simulink model "ModelNonLinearMechFram"  (R2014b)
settings: Solver=ode45  StartTime=0.0  StopTime=1.5  FixedStep=0.001  RelTol=1e-3
InitFcn:
  | InitModel;
values from neighbouring files (symbols this model uses):
  R1 = 1.8e3    (= 1800)    [InitModel.m]    (also in SystemModel.m; SystemModel_marco.m)
  R4 = 47e3    (= 47000)    [InitModel.m]    (also in SystemModel.m; SystemModel_marco.m)
  R6 = 100e3    (= 100000)    [InitModel.m]    (also in SystemModel.m; SystemModel_marco.m)
  R7 = 27e3    (= 27000)    [InitModel.m]    (also in SystemModel.m; SystemModel_marco.m)
  rad2rpm = 60/(2*pi)    (= 9.54929658551)    [InitModel.m]    (also in SystemModel.m)
  Rs = 0.1    [InitModel.m]    (also in SystemModel.m; SystemModel_marco.m)
  Rv2 = realp('Rv2', 0)    [InitModel.m]    (also in SystemModel.m = realp('Rv2', 10000); SystemModel_marco.m = 0)
  Vdc = 30/8    (= 3.75)    [InitModel.m]    (also in SystemModel.m = 30; SystemModel_marco.m = 30)
  Vsat = 10    [InitModel.m]
undefined symbols (not defined in the file or in its folder): motor, pid, sigbuilder_block
libraries: cstblocks x5, simulink x1
settings Model: Creator=Edoardo  LastModifiedBy=Edoardo
settings SolverCC: ZeroCrossAlgorithm=Adaptive

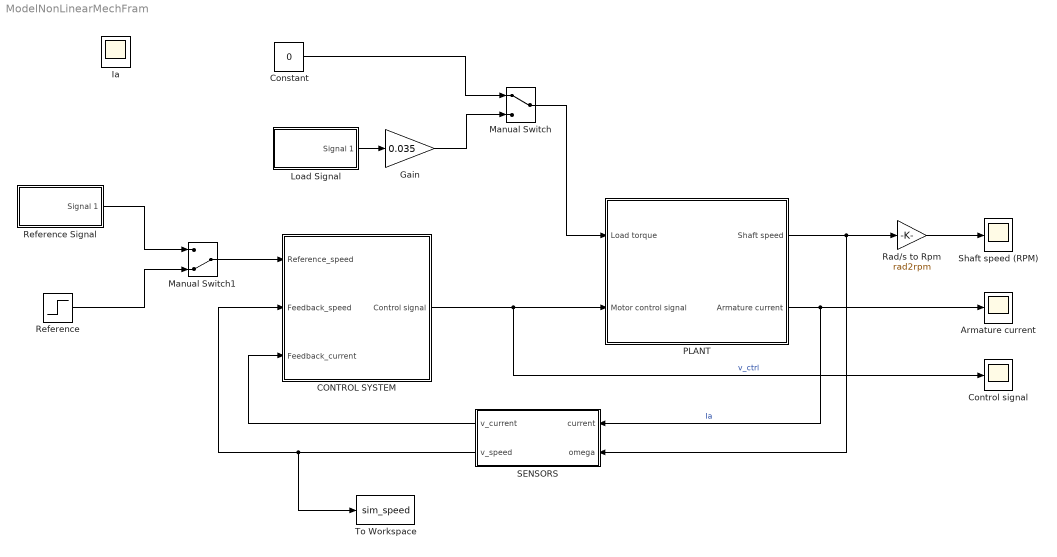
== system ModelNonLinearMechFram ==
  "Armature current " : Scope
      settings: YMin=-0.2  YMax=1.4  SaveName=ScopeData3
  CONTROL SYSTEM : Subsystem
  Constant : Constant  Value=0
  Control signal : Scope
      settings: YMin=-0.2  YMax=1.4  SaveName=ScopeData5
  Gain : Gain  Gain=0.035
  Load Signal : Subsystem  Tag=STV Subsys  LoadFcn=sigbuilder_block('load');  StartFcn=sigbuilder_block('start');  StopFcn=sigbuilder_block('stop');  ClipboardFcn=sigbuilder_block('clipboard');  mask(Sigbuilder block){}
      mask help: Simulink:masks:SigbuilderBlock_MD
      mask init:
      | if ~strcmp(get_param(bdroot(gcbh),'SimulationStatus'),'stopped') tuvar = sigbuilder_block('maskInit'); end
      settings: CopyFcn=sigbuilder_block('copy');  DeleteFcn=sigbuilder_block('delete');  ModelCloseFcn=sigbuilder_block('modelClose');  PreSaveFcn=sigbuilder_block('preSave');  PauseFcn=sigbuilder_block('pause');  ContinueFcn=sigbuilder_block('continue');  NameChangeFcn=sigbuilder_block('namechange');  OpenFcn=sigbuilder_block('open',[437.6 199.2 550.4 400 ]);  CloseFcn=sigbuilder_block('close');
      mask Display: plot(0, 0, 100, 100,[2, 2, 32, 32, 2], [68, 8, 8, 68, 68],[32, 2], [38, 38], [32, 19, 2],[53, 60, 44], [32, 17, 17, 2],[16, 16, 31, 31]);txt = getActiveGroup(gcbh);text(2, 100, txt,'verticalAlignment', 'top');
  Manual Switch : ManualSwitch
  Manual Switch1 : ManualSwitch  CurrentSetting=0
  PLANT : Subsystem
  Rad/s to Rpm : Gain  Gain=rad2rpm
  Reference : Step  Time=0.5  After=8  SampleTime=0
  Reference Signal : Subsystem  Tag=STV Subsys  LoadFcn=sigbuilder_block('load');  StartFcn=sigbuilder_block('start');  StopFcn=sigbuilder_block('stop');  ClipboardFcn=sigbuilder_block('clipboard');  mask(Sigbuilder block){}
      mask help: Simulink:masks:SigbuilderBlock_MD
      mask init:
      | if ~strcmp(get_param(bdroot(gcbh),'SimulationStatus'),'stopped') tuvar = sigbuilder_block('maskInit'); end
      settings: CopyFcn=sigbuilder_block('copy');  DeleteFcn=sigbuilder_block('delete');  ModelCloseFcn=sigbuilder_block('modelClose');  PreSaveFcn=sigbuilder_block('preSave');  PauseFcn=sigbuilder_block('pause');  ContinueFcn=sigbuilder_block('continue');  NameChangeFcn=sigbuilder_block('namechange');  OpenFcn=sigbuilder_block('open',[437.6 199.2 550.4 400 ]);  CloseFcn=sigbuilder_block('close');
      mask Display: plot(0, 0, 100, 100,[2, 2, 32, 32, 2], [68, 8, 8, 68, 68],[32, 2], [38, 38], [32, 19, 2],[53, 60, 44], [32, 17, 17, 2],[16, 16, 31, 31]);txt = getActiveGroup(gcbh);text(2, 100, txt,'verticalAlignment', 'top');
  SENSORS : Subsystem
  Shaft speed (RPM) : Scope
      settings: TimeRange=1.5  YMin=-1000  YMax=7000
  To Workspace : ToWorkspace  VariableName=sim_speed  SaveFormat=Timeseries  SampleTime=-1
      settings: Save2DSignal=2-D array (concatenate along first dimension)
  Ia : Scope
  wires:
  Rad/s to Rpm/1 -> Shaft speed (RPM)/1
  PLANT/1(Shaft speed) -> SENSORS/2(omega), Rad/s to Rpm/1
  CONTROL SYSTEM/1(Control signal) -> Control signal/1, PLANT/2(Motor control signal)  "v_ctrl"
  PLANT/2(Armature current) -> SENSORS/1(current), "Armature current "/1  "Ia"
  SENSORS/2(v_speed) -> To Workspace/1, CONTROL SYSTEM/2(Feedback_speed)
  SENSORS/1(v_current) -> CONTROL SYSTEM/3(Feedback_current)
  Manual Switch/1 -> PLANT/1(Load torque)
  Constant/1 -> Manual Switch/1
  Load Signal/1(Signal 1) -> Gain/1
  Gain/1 -> Manual Switch/2
  Manual Switch1/1 -> CONTROL SYSTEM/1(Reference_speed)
  Reference Signal/1(Signal 1) -> Manual Switch1/1
  Reference/1 -> Manual Switch1/2

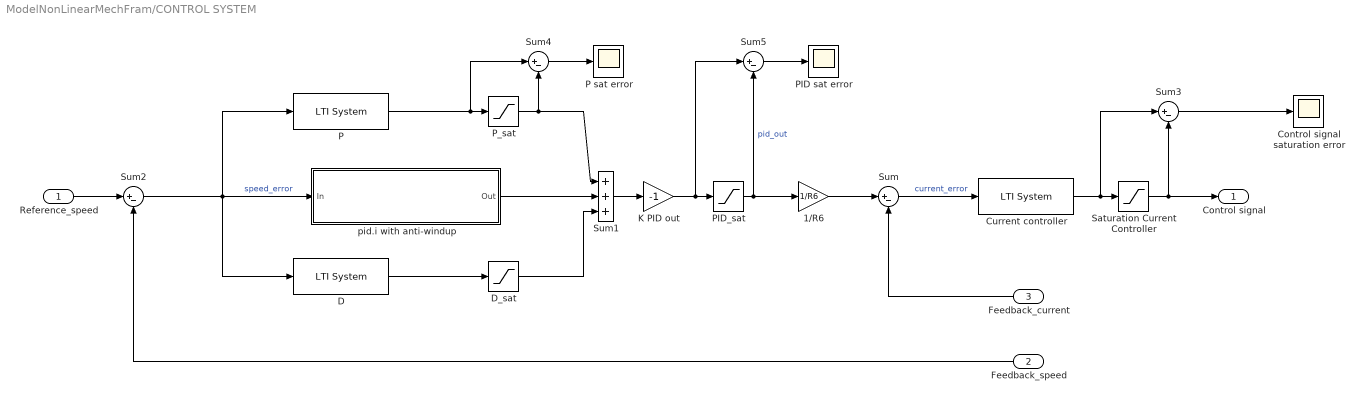
== system ModelNonLinearMechFram/CONTROL SYSTEM ==
  Reference_speed : Inport
  Feedback_speed : Inport  Port=2
  Feedback_current : Inport  Port=3
  1/R6 : Gain  Gain=1/R6
  Control signal saturation error : Scope
      settings: SaveName=ScopeData4  Decimation=10
  Current controller : cstblocks/LTI System  sys=C1  IC=[]
  D : cstblocks/LTI System  sys=pid.d  IC=[]
  D_sat : Saturate  UpperLimit=Vsat  LowerLimit=-Vsat
  K PID out : Gain  Gain=-1
  P : cstblocks/LTI System  sys=pid.p  IC=[]
  P sat error : Scope
      settings: SaveName=ScopeData6  Decimation=10
  PID sat error : Scope
      settings: SaveName=ScopeData8  Decimation=10
  PID_sat : Saturate  UpperLimit=9.1  LowerLimit=-9.1
  P_sat : Saturate  UpperLimit=Vsat  LowerLimit=-Vsat
  Saturation Current Controller : Saturate  UpperLimit=Vsat  LowerLimit=-Vsat
  Sum{,2..5} (5 alike) : Sum  Inputs=|+-
  Sum1 : Sum  Inputs=+++
  pid.i with anti-windup : Subsystem
  Control signal : Outport
  wires:
  1/R6/1 -> Sum/1
  Current controller/1 -> Sum3/1, Saturation Current Controller/1
  Sum/1 -> Current controller/1  "current_error"
  Feedback_current/1 -> Sum/2
  Saturation Current Controller/1 -> Control signal/1, Sum3/2
  D/1 -> D_sat/1
  D_sat/1 -> Sum1/3
  PID_sat/1 -> 1/R6/1, Sum5/2  "pid_out"
  Sum1/1 -> K PID out/1
  Reference_speed/1 -> Sum2/1
  Feedback_speed/1 -> Sum2/2
  Sum2/1 -> pid.i with anti-windup/1(In), P/1, D/1  "speed_error"
  pid.i with anti-windup/1(Out) -> Sum1/2
  Sum3/1 -> Control signal saturation error/1
  P/1 -> Sum4/1, P_sat/1
  P_sat/1 -> Sum4/2, Sum1/1
  Sum4/1 -> P sat error/1
  K PID out/1 -> Sum5/1, PID_sat/1
  Sum5/1 -> PID sat error/1

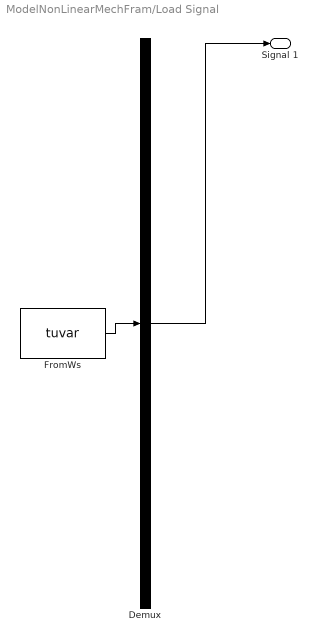
== system ModelNonLinearMechFram/Load Signal ==
  Demux : Demux  Tag=STV Demux  Outputs=1
  FromWs : FromWorkspace  Tag=STV FromWs  VariableName=tuvar  SampleTime=0
      SigBuilderData=|
      | common.afterFinalStr = 'Extrapolate'
      | common.sampleTime = 0
      | dataSet.timeRange = [0 10]
      | dataSet.name = 'Group 1'
      | sbobj.Groups.Name = 'Group 1'
      | sbobj.Groups.Signals.Name = 'Signal 1'
      | sbobj.Groups.Signals.XData = [0 0.1 0.3 6 6 10]
      | sbobj.Groups.Signals.YData = [0 0 1 1 0 0]
  Signal 1 : Outport  Tag=STV Outport
  wires:
  Demux/1 -> Signal 1/1
  FromWs/1 -> Demux/1

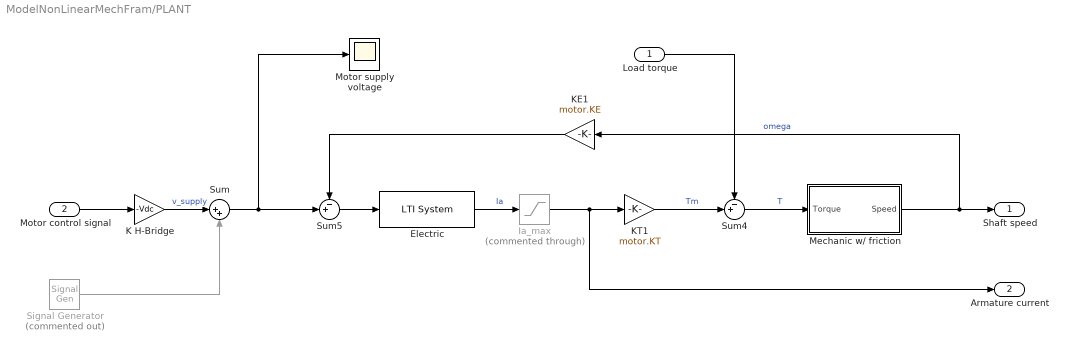
== system ModelNonLinearMechFram/PLANT ==
  Load torque : Inport
  Motor control signal : Inport  Port=2
  Electric : cstblocks/LTI System  sys=G1  IC=[]
  Ia_max : Saturate  Commented=through  UpperLimit=motor.Ia_max  LowerLimit=-motor.Ia_max
  K H-Bridge : Gain  Gain=-Vdc
  KE1 : Gain  Gain=motor.KE
  KT1 : Gain  Gain=motor.KT
  Mechanic w/ friction : Subsystem
  Motor supply voltage : Scope
      settings: SaveName=ScopeData2
  Signal Generator : SignalGenerator  Commented=on  WaveForm=square  Amplitude=0.03  Frequency=23e3
  Sum : Sum  Inputs=|++
  Sum4 : Sum  Inputs=-+|
  Sum5 : Sum  Inputs=-+|
  Shaft speed : Outport
  Armature current : Outport  Port=2
  wires:
  Electric/1 -> Ia_max/1  "Ia"
  Sum4/1 -> Mechanic w/ friction/1(Torque)  "T"
  Motor control signal/1 -> K H-Bridge/1
  Sum5/1 -> Electric/1
  Mechanic w/ friction/1(Speed) -> Shaft speed/1, KE1/1  "omega"
  KE1/1 -> Sum5/1
  Ia_max/1 -> KT1/1, Armature current/1
  Load torque/1 -> Sum4/1
  KT1/1 -> Sum4/2  "Tm"
  K H-Bridge/1 -> Sum/1  "v_supply"
  Signal Generator/1 -> Sum/2
  Sum/1 -> Motor supply voltage/1, Sum5/2

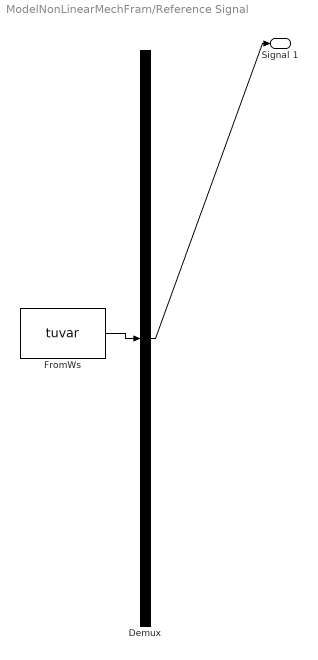
== system ModelNonLinearMechFram/Reference Signal ==
  Demux : Demux  Tag=STV Demux  Outputs=1
  FromWs : FromWorkspace  Tag=STV FromWs  VariableName=tuvar  SampleTime=0
      SigBuilderData=|
      | common.afterFinalStr = 'Extrapolate'
      | common.sampleTime = 0
      | dataSet.timeRange = [0 10]
      | dataSet.name = 'Group 1'
      | sbobj.Groups.Name = 'Group 1'
      | sbobj.Groups.Signals.Name = 'Signal 1'
      | sbobj.Groups.Signals.XData = [0 0.2 0.2 10]
      | sbobj.Groups.Signals.YData = [1.6 1.6 2.4 2.4]
  Signal 1 : Outport  Tag=STV Outport
  wires:
  FromWs/1 -> Demux/1
  Demux/1 -> Signal 1/1

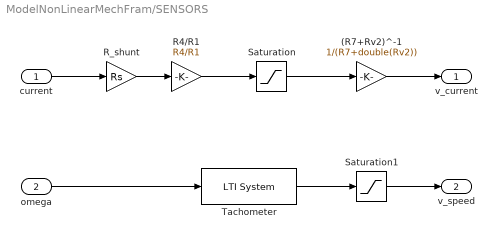
== system ModelNonLinearMechFram/SENSORS ==
  current : Inport
  omega : Inport  Port=2
  (R7+Rv2)^-1 : Gain  Gain=1/(R7+double(Rv2))
  R4/R1 : Gain  Gain=R4/R1
  R_shunt : Gain  Gain=Rs
  Saturation : Saturate  UpperLimit=Vsat  LowerLimit=-Vsat
  Saturation1 : Saturate  UpperLimit=Vsat  LowerLimit=-Vsat
  Tachometer : cstblocks/LTI System  sys=H2  IC=[]
  v_current : Outport
  v_speed : Outport  Port=2
  wires:
  Tachometer/1 -> Saturation1/1
  R4/R1/1 -> Saturation/1
  current/1 -> R_shunt/1
  omega/1 -> Tachometer/1
  (R7+Rv2)^-1/1 -> v_current/1
  R_shunt/1 -> R4/R1/1
  Saturation/1 -> (R7+Rv2)^-1/1
  Saturation1/1 -> v_speed/1

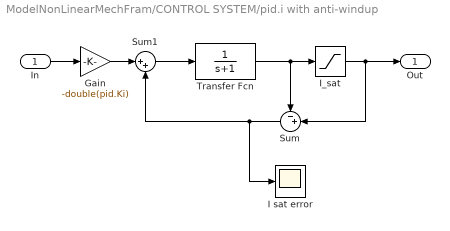
== system ModelNonLinearMechFram/CONTROL SYSTEM/pid.i with anti-windup ==
  In : Inport
  Gain : Gain  Gain=-double(pid.Ki)
  I sat error : Scope
      settings: SaveName=ScopeData7  Decimation=10
  I_sat : Saturate  UpperLimit=Vsat  LowerLimit=-Vsat
  Sum : Sum  Inputs=-+|
  Sum1 : Sum  Inputs=|++
  Transfer Fcn : TransferFcn  Denominator=[1 1]
  Out : Outport
  wires:
  I_sat/1 -> Sum/2, Out/1
  Transfer Fcn/1 -> Sum/1, I_sat/1
  In/1 -> Gain/1
  Sum1/1 -> Transfer Fcn/1
  Sum/1 -> Sum1/2, I sat error/1
  Gain/1 -> Sum1/1

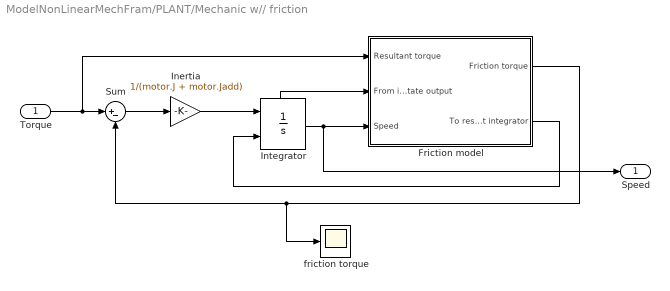
== system ModelNonLinearMechFram/PLANT/Mechanic w// friction ==
  Torque : Inport
  Friction model : Subsystem
  Inertia : Gain  Gain=1/(motor.J + motor.Jadd)
  Integrator : Integrator  ExternalReset=rising  ShowStatePort=on
  Sum : Sum  Inputs=|+-
  friction torque : Scope
      settings: SaveName=ScopeData9
  Speed : Outport
  wires:
  Torque/1 -> Friction model/1(Resultant torque), Sum/1
  Inertia/1 -> Integrator/1
  Friction model/1(Friction torque) -> friction torque/1, Sum/2
  Integrator/State -> Friction model/2(From integrator state output)
  Integrator/1 -> Speed/1, Friction model/3(Speed)
  Sum/1 -> Inertia/1
  Friction model/2(To reset integrator) -> Integrator/2

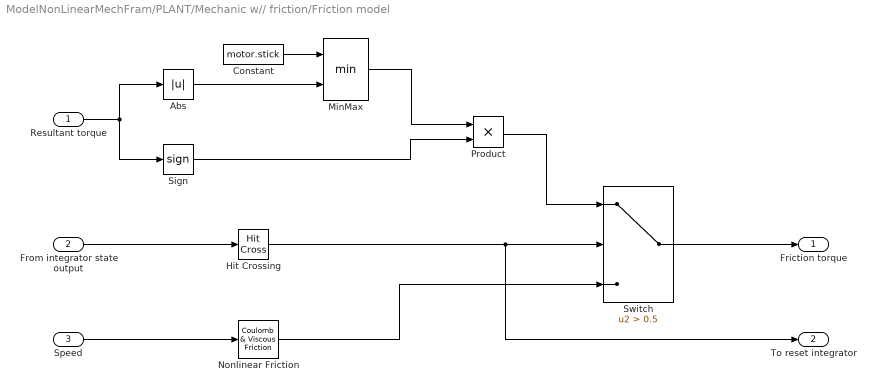
== system ModelNonLinearMechFram/PLANT/Mechanic w// friction/Friction model ==
  Resultant torque : Inport
  From integrator state output : Inport  Port=2
  Speed : Inport  Port=3
  Abs : Abs
  Constant : Constant  Value=motor.stick
  Hit Crossing : HitCross
  MinMax : MinMax  Inputs=2
  Nonlinear Friction : simulink/Discontinuities/Coulomb & Viscous Friction  offset=motor.coulomb  gain=motor.beta
  Product : Product
  Sign : Signum
  Switch : Switch  Criteria=u2 > Threshold  Threshold=0.5
  Friction torque : Outport
  To reset integrator : Outport  Port=2
  wires:
  MinMax/1 -> Product/1
  Constant/1 -> MinMax/1
  Sign/1 -> Product/2
  Abs/1 -> MinMax/2
  Product/1 -> Switch/1
  From integrator state output/1 -> Hit Crossing/1
  Switch/1 -> Friction torque/1
  Resultant torque/1 -> Sign/1, Abs/1
  Hit Crossing/1 -> To reset integrator/1, Switch/2
  Speed/1 -> Nonlinear Friction/1
  Nonlinear Friction/1 -> Switch/3
